simulink model "mavsim_chap11"  (R2019a)
settings: Solver=ode45  StartTime=0.0  StopTime=150  RelTol=1e-3  EnableMultiTasking=on
InitFcn:
  | clear all
  | path(pathdef)
  | addpath('../chap2')
  | addpath('../parameters/')
  | aerosonde_parameters
  | simulation_parameters
  | wind_parameters
  | sensor_parameters
  | addpath('../chap3')
  | addpath('../chap4')
  | addpath('../chap6')
  | compute_autopilot_gains
  | addpath('../chap7')
  | addpath('../chap8')
  | addpath('../chap10')
  | addpath('../chap11')
  | planner_parameters
undefined symbols (not defined in the file or in its folder): autopilot, drawEnvironment_chap11, forces_moments, P, path_follow, path_manager, path_planner_chap11, PLAN, SIM, true_states
libraries: simulink x3
settings Model: Creator=beard  LastModifiedBy=Hugo Pereira
settings DataIOCC: LimitDataPoints=on  SaveFormat=Array  SignalLoggingSaveFormat=ModelDataLogs  ReturnWorkspaceOutputs=off
settings OptimizationCC: ExpressionDepthLimit=2147483647  InitFltsAndDblsToZero=on  LifeSpan=inf
settings DebuggingCC: UnderspecifiedInitializationDetection=Classic  MergeDetectMultiDrivingBlocksExec=none  SolverPrmCheckMsg=warning  FcnCallInpInsideContextMsg=warning  AllowSymbolicDim=off  StateNameClashWarn=warning  SFUnexpectedBacktrackingDiag=warning  SFNoUnconditionalDefaultTransitionDiag=warning  SFExecutionAtInitializationDiag=none  ArithmeticOperatorsInVariantConditions=warning
settings HardwareCC: ProdBitPerPointer=32  ProdBitPerSizeT=32  ProdBitPerPtrDiffT=32  ProdLargestAtomicFloat=None  ProdIntDivRoundTo=Undefined  ProdEndianess=Unspecified  ProdWordSize=32  ProdHWDeviceType=32-bit Generic
settings ModelReferenceCC: PropagateSignalLabelsOutOfModel=off
settings SFSimCC: SimUseLocalCustomCode=off  SimParseCustomCode=off
settings RTWCC: RTWUseLocalCustomCode=off
settings CodeAppCC: StateflowObjectComments=on
settings GRTTargetCC: TargetLangStandard=C89/C90 (ANSI)  GeneratePreprocessorConditionals=Disable all  CombineOutputUpdateFcns=off  GRTInterface=on
settings ConfigComp: CovMetricSettings=dw  CovHtmlReporting=on  CovSaveCumulativeToWorkspaceVar=on  CovSaveSingleToWorkspaceVar=on  CovExternalEMLEnable=off  CovSFcnEnable=off

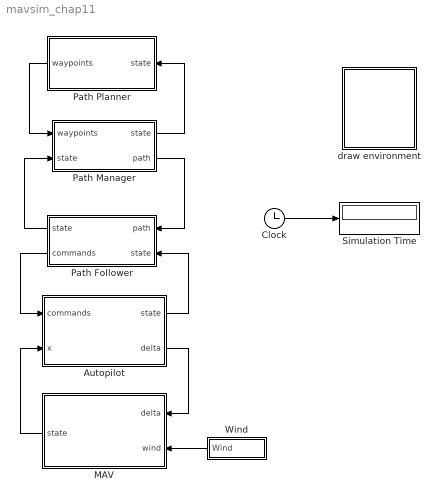
== system mavsim_chap11 ==
  Autopilot : Subsystem
      mask Display: image(imread('../autopilot/simulink_imgs/kestrel.jpg'));
  Clock : Clock
  MAV : Subsystem
      mask Display: image(imread('../autopilot/simulink_imgs/batcam.png'));
  Path Follower : Subsystem
  Path Manager : Subsystem
  Path Planner : Subsystem
  Simulation Time : Display
  Wind : Subsystem
  draw environment : Subsystem
      mask Display: image(imread('tv.jpg'))
  wires:
  Clock/1 -> Simulation Time/1
  Path Planner/1(waypoints) -> Path Manager/1(waypoints)
  Path Manager/1("state ") -> Path Planner/1(state)
  Path Follower/1("state ") -> Path Manager/2(state)
  Path Manager/2(path) -> Path Follower/1(path)
  Path Follower/2(commands) -> Autopilot/1(commands)
  Wind/1(Wind) -> MAV/2(wind)
  Autopilot/2(delta) -> MAV/1(delta)
  MAV/1(state) -> Autopilot/2(x)
  Autopilot/1(state) -> Path Follower/2(state)

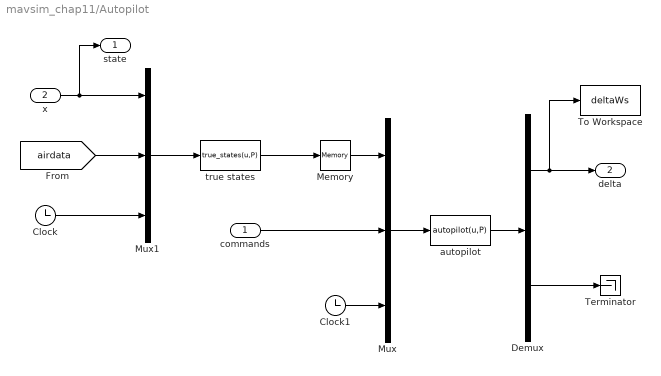
== system mavsim_chap11/Autopilot ==
  commands : Inport
  x : Inport  Port=2
  Clock : Clock
  Clock1 : Clock
  Demux : Demux  Outputs=[4;2]
  Memory : Memory
  Mux : Mux  Inputs=3
  Mux1 : Mux  Inputs=3
  Terminator : Terminator
  To Workspace : ToWorkspace  VariableName=deltaWs  SampleTime=-1
  autopilot : MATLABFcn  MATLABFcn=autopilot(u,P)  OutputDimensions=4+2  SampleTime=P.Ts
  true states : MATLABFcn  MATLABFcn=true_states(u,P)  OutputDimensions=19  SampleTime=P.Ts
  state : Outport
  delta : Outport  Port=2
  wires:
  Mux/1 -> autopilot/1
  Clock/1 -> Mux1/3
  autopilot/1 -> Demux/1
  Demux/1 -> To Workspace/1, delta/1
  Demux/2 -> Terminator/1
  commands/1 -> Mux/2
  Mux1/1 -> true states/1
  x/1 -> state/1, Mux1/1
  true states/1 -> Memory/1
  [airdata] -> Mux1/2
  Memory/1 -> Mux/1
  Clock1/1 -> Mux/3

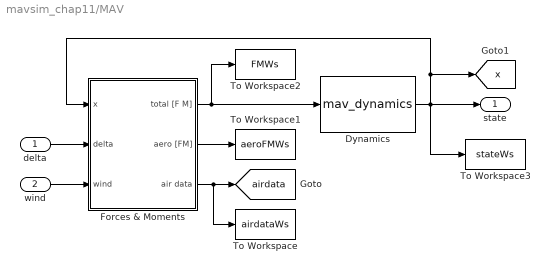
== system mavsim_chap11/MAV ==
  delta : Inport
  wind : Inport  Port=2
  Dynamics : S-Function  FunctionName=mav_dynamics  Parameters=P  SFunctionDeploymentMode=off  EnableBusSupport=off
  Forces & Moments : Subsystem
  To Workspace : ToWorkspace  VariableName=airdataWs  SampleTime=-1
  To Workspace1 : ToWorkspace  VariableName=aeroFMWs  SampleTime=-1
  To Workspace2 : ToWorkspace  VariableName=FMWs  SampleTime=-1
  To Workspace3 : ToWorkspace  VariableName=stateWs  SampleTime=-1
  state : Outport
  tag scope: airdata=global, x=global
  wires:
  Dynamics/1 -> Forces & Moments/1(x), [x], To Workspace3/1, state/1
  Forces & Moments/1(total [F M]) -> To Workspace2/1, Dynamics/1
  Forces & Moments/3(air data) -> [airdata], To Workspace/1
  delta/1 -> Forces & Moments/2(delta)
  wind/1 -> Forces & Moments/3(wind)
  Forces & Moments/2(aero [FM]) -> To Workspace1/1

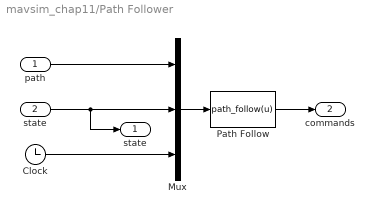
== system mavsim_chap11/Path Follower ==
  path : Inport
  state : Inport  Port=2
  Clock : Clock
  Mux : Mux  Inputs=3
  Path Follow : MATLABFcn  MATLABFcn=path_follow(u)  OutputDimensions=4  SampleTime=P.Ts
  "state " : Outport
  commands : Outport  Port=2
  wires:
  Path Follow/1 -> commands/1
  Mux/1 -> Path Follow/1
  path/1 -> Mux/1
  Clock/1 -> Mux/3
  state/1 -> Mux/2, "state "/1

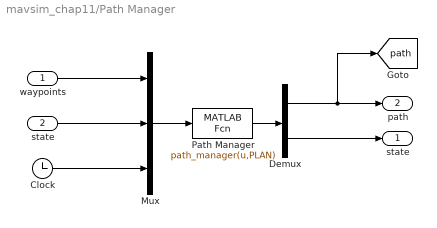
== system mavsim_chap11/Path Manager ==
  waypoints : Inport
  state : Inport  Port=2
  Clock : Clock
  Demux : Demux  Outputs=[13;17]
  Mux : Mux  Inputs=3
  Path Manager : MATLABFcn  MATLABFcn=path_manager(u,PLAN)  OutputDimensions=30  SampleTime=P.Ts
  "state " : Outport
  path : Outport  Port=2
  tag scope: path=global
  wires:
  Demux/2 -> "state "/1
  Demux/1 -> [path], path/1
  Path Manager/1 -> Demux/1
  waypoints/1 -> Mux/1
  state/1 -> Mux/2
  Clock/1 -> Mux/3
  Mux/1 -> Path Manager/1

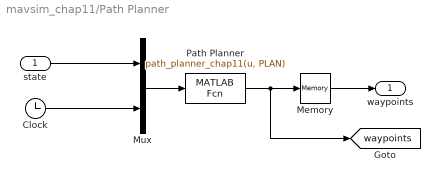
== system mavsim_chap11/Path Planner ==
  state : Inport
  Clock : Clock
  Memory : Memory
  Mux : Mux  Inputs=2
  Path Planner : MATLABFcn  MATLABFcn=path_planner_chap11(u, PLAN)  OutputDimensions=1+5*PLAN.size_waypoint_array  SampleTime=100*P.Ts
  waypoints : Outport
  tag scope: waypoints=global
  wires:
  Mux/1 -> Path Planner/1
  Clock/1 -> Mux/2
  state/1 -> Mux/1
  Path Planner/1 -> Memory/1, [waypoints]
  Memory/1 -> waypoints/1

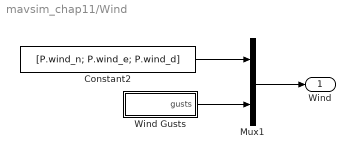
== system mavsim_chap11/Wind ==
  Constant2 : Constant  Value=[P.wind_n; P.wind_e; P.wind_d]
  Mux1 : Mux  Inputs=2
  Wind Gusts : Subsystem
  Wind : Outport
  wires:
  Constant2/1 -> Mux1/1
  Mux1/1 -> Wind/1
  Wind Gusts/1(gusts) -> Mux1/2

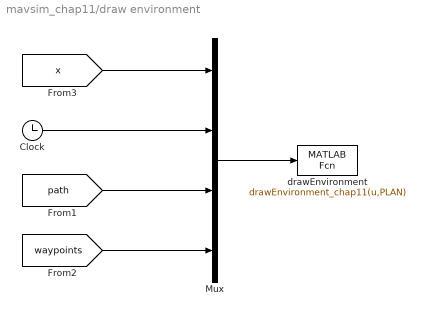
== system mavsim_chap11/draw environment ==
  Clock : Clock
  Mux : Mux
  drawEnvironment : MATLABFcn  MATLABFcn=drawEnvironment_chap11(u,PLAN)  OutputDimensions=0  SampleTime=SIM.ts_plotting
  wires:
  Clock/1 -> Mux/2
  [x] -> Mux/1
  Mux/1 -> drawEnvironment/1
  [path] -> Mux/3
  [waypoints] -> Mux/4

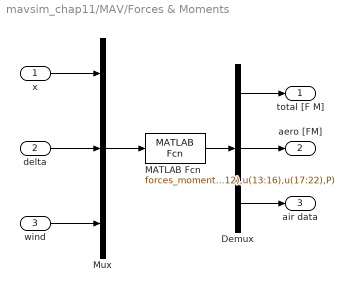
== system mavsim_chap11/MAV/Forces & Moments ==
  x : Inport
  delta : Inport  Port=2
  wind : Inport  Port=3
  Demux : Demux  Outputs=[6;6;7]
  MATLAB Fcn : MATLABFcn  MATLABFcn=forces_moments(u(1:12),u(13:16),u(17:22),P)  OutputDimensions=19
  Mux : Mux  Inputs=3
  total [F M] : Outport
  aero [FM] : Outport  Port=2
  air data : Outport  Port=3
  wires:
  Mux/1 -> MATLAB Fcn/1
  Demux/1 -> total [F M]/1
  MATLAB Fcn/1 -> Demux/1
  wind/1 -> Mux/3
  delta/1 -> Mux/2
  x/1 -> Mux/1
  Demux/3 -> air data/1
  Demux/2 -> aero [FM]/1

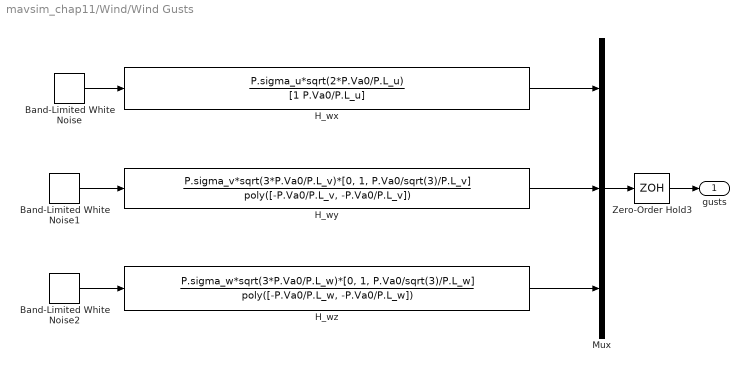
== system mavsim_chap11/Wind/Wind Gusts ==
  Band-Limited White Noise : simulink/Sources/Band-Limited White Noise  Cov=[1]  Ts=P.Ts  seed=[23341]
  Band-Limited White Noise1 : simulink/Sources/Band-Limited White Noise  Cov=[1]  Ts=P.Ts  seed=[23341]
  Band-Limited White Noise2 : simulink/Sources/Band-Limited White Noise  Cov=[1]  Ts=P.Ts  seed=[23341]
  H_wx : TransferFcn  Numerator=P.sigma_u*sqrt(2*P.Va0/P.L_u)  Denominator=[1 P.Va0/P.L_u]
  H_wy : TransferFcn  Numerator=P.sigma_v*sqrt(3*P.Va0/P.L_v)*[0, 1, P.Va0/sqrt(3)/P.L_v]  Denominator=poly([-P.Va0/P.L_v, -P.Va0/P.L_v])
  H_wz : TransferFcn  Numerator=P.sigma_w*sqrt(3*P.Va0/P.L_w)*[0, 1, P.Va0/sqrt(3)/P.L_w]  Denominator=poly([-P.Va0/P.L_w, -P.Va0/P.L_w])
  Mux : Mux  Inputs=3
  Zero-Order Hold3 : ZeroOrderHold  SampleTime=P.Ts
  gusts : Outport
  wires:
  H_wx/1 -> Mux/1
  Band-Limited White Noise/1 -> H_wx/1
  H_wy/1 -> Mux/2
  Band-Limited White Noise1/1 -> H_wy/1
  H_wz/1 -> Mux/3
  Band-Limited White Noise2/1 -> H_wz/1
  Mux/1 -> Zero-Order Hold3/1
  Zero-Order Hold3/1 -> gusts/1
